simulink model "task5_lab13"  (R2021a)
settings: Solver=VariableStepAuto  StartTime=0.0  StopTime=10.0  RelTol=1e-3
settings Model: Creator=reemb  LastModifiedBy=reemb

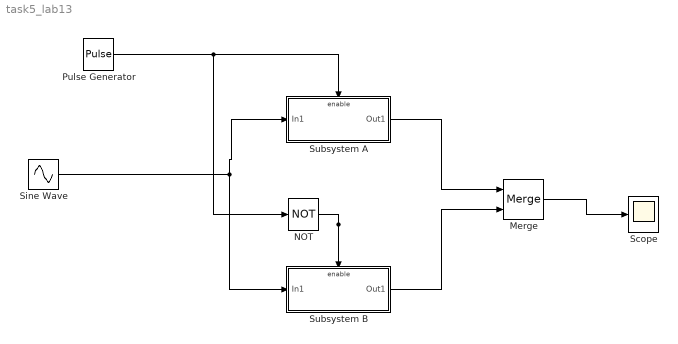
== system task5_lab13 ==
  Merge : Merge
  NOT : Logic  Operator=NOT  AllPortsSameDT=off  OutDataTypeStr=boolean
  Pulse Generator : DiscretePulseGenerator  PulseType=Time based  Period=10  PulseWidth=5
  Scope : Scope
  Sine Wave : Sin  SampleTime=0
  Subsystem A : Subsystem  TreatAsAtomicUnit=on
  Subsystem B : Subsystem  TreatAsAtomicUnit=on
  wires:
  Sine Wave/1 -> Subsystem A/1(In1), Subsystem B/1(In1)
  Pulse Generator/1 -> NOT/1, Subsystem A/Enable
  NOT/1 -> Subsystem B/Enable
  Merge/1 -> Scope/1
  Subsystem A/1(Out1) -> Merge/1
  Subsystem B/1(Out1) -> Merge/2

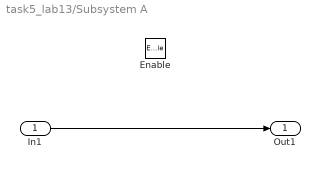
== system task5_lab13/Subsystem A ==
  In1 : Inport
  Enable : EnablePort
  Out1 : Outport
  wires:
  In1/1 -> Out1/1

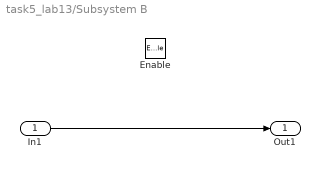
== system task5_lab13/Subsystem B ==
  In1 : Inport
  Enable : EnablePort
  Out1 : Outport
  wires:
  In1/1 -> Out1/1
